simulink model "task8_simulink_backup_lineare"  (R2024b)
settings: Solver=VariableStepAuto  StartTime=0.0  StopTime=10.0  RelTol=1e-3
values from neighbouring files (symbols this model uses):
  A = [ ... (first row only)    [longitudinal_linear_model.m]
  alpha_trim = trim_solution(2)    [main.m]
  B = [ ... (first row only)    [longitudinal_linear_model.m]
  h_trim = 0    [main.m]
  x_trim = [ ... (first row only)    [main.m]
settings Model: Creator=Admin  LastModifiedBy=Admin

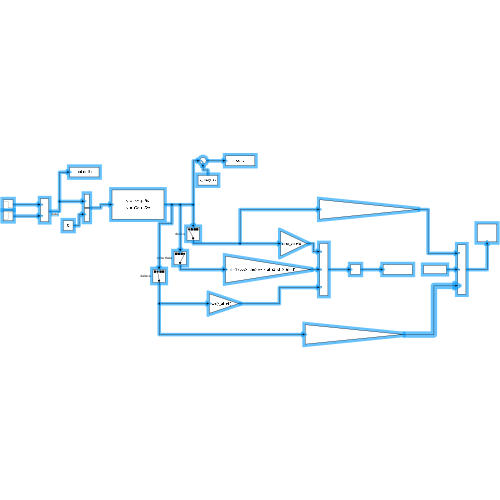
[thumbnail: Simulink's stored preview of the top-level diagram]
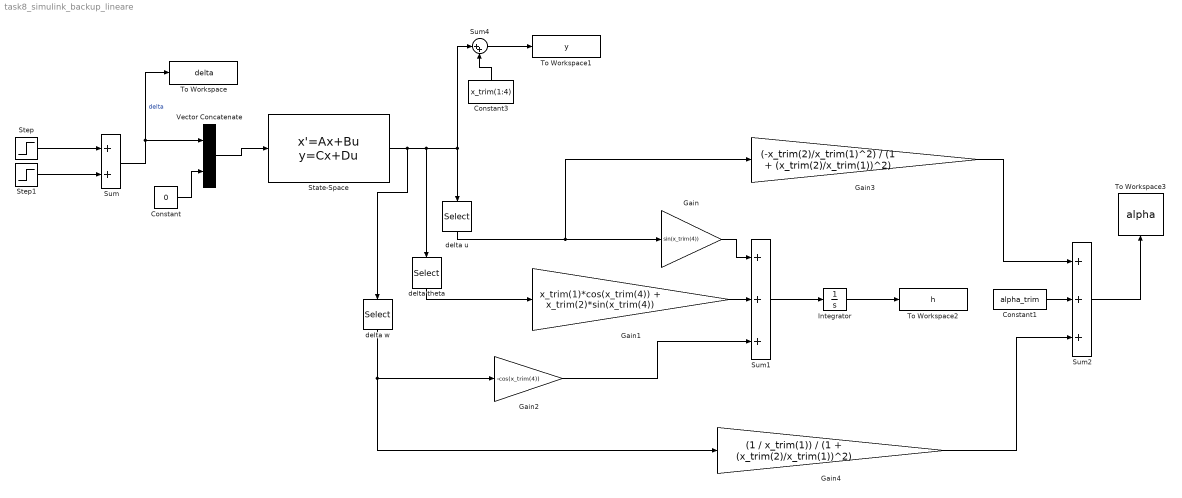
== system task8_simulink_backup_lineare ==
  Constant : Constant  Value=0
  Constant1 : Constant  Value=alpha_trim
  Constant3 : Constant  Value=x_trim(1:4)
  Gain : Gain  Gain=sin(x_trim(4))
  Gain1 : Gain  Gain=x_trim(1)*cos(x_trim(4)) + x_trim(2)*sin(x_trim(4))
  Gain2 : Gain  Gain=-cos(x_trim(4))
  Gain3 : Gain  Gain=(-x_trim(2)/x_trim(1)^2) / (1 + (x_trim(2)/x_trim(1))^2)
  Gain4 : Gain  Gain=(1 / x_trim(1)) / (1 + (x_trim(2)/x_trim(1))^2)
  Integrator : Integrator  InitialCondition=h_trim
  State-Space : StateSpace  A=A  B=B  C=eye(4)  D=zeros(4,2)  InitialCondition=zeros(4,1)
  Step : Step  Time=5  After=- pi/180  SampleTime=0
  Step1 : Step  Time=10  After=(pi/180)  SampleTime=0
  Sum : Sum
  Sum1 : Sum  Inputs=+++
  Sum2 : Sum  Inputs=+++
  Sum4 : Sum  Inputs=|++
  To Workspace : ToWorkspace  VariableName=delta  SampleTime=-1
  To Workspace1 : ToWorkspace  VariableName=y  SaveFormat=Structure  SampleTime=-1
      settings: Save2DSignal=2-D array (concatenate along first dimension)
  To Workspace2 : ToWorkspace  VariableName=h  SampleTime=-1
  To Workspace3 : ToWorkspace  VariableName=alpha  SampleTime=-1
  Vector Concatenate : Concatenate
  delta theta : Selector  InputPortWidth=4  IndexOptions=Index vector (dialog)  Indices=4  OutputSizes=1
  delta u : Selector  InputPortWidth=4  IndexOptions=Index vector (dialog)  Indices=1  OutputSizes=1
  delta w : Selector  InputPortWidth=4  IndexOptions=Index vector (dialog)  Indices=2  OutputSizes=1
  wires:
  Gain1/1 -> Sum1/2
  Sum2/1 -> To Workspace3/1
  Sum4/1 -> To Workspace1/1
  Constant1/1 -> Sum2/2
  Gain/1 -> Sum1/1
  Sum1/1 -> Integrator/1
  delta theta/1 -> Gain1/1
  Constant3/1 -> Sum4/2
  Gain2/1 -> Sum1/3
  Step/1 -> Sum/1
  Sum/1 -> Vector Concatenate/1, To Workspace/1  "delta"
  Constant/1 -> Vector Concatenate/2
  State-Space/1 -> delta theta/1, Sum4/1, delta u/1, delta w/1
  Vector Concatenate/1 -> State-Space/1
  Step1/1 -> Sum/2
  Gain3/1 -> Sum2/1
  delta u/1 -> Gain3/1, Gain/1
  delta w/1 -> Gain4/1, Gain2/1
  Integrator/1 -> To Workspace2/1
  Gain4/1 -> Sum2/3
